simulink model "Continuous_Model"  (R2021b)
settings: Solver=VariableStepAuto  StartTime=0.0  StopTime=200.0  RelTol=1e-3
values from neighbouring files (symbols this model uses):
  mu0 = 0    [Continuous_Model_Parameters.m]
  n0 = 0    [Continuous_Model_Parameters.m]
  r0 = 0    [Continuous_Model_Parameters.m]
  s0 = 5    [Continuous_Model_Parameters.m]
  str0 = 0    [Continuous_Model_Parameters.m]
  T0 = 1    [Continuous_Model_Parameters.m]
  vx0 = 5    [Continuous_Model_Parameters.m]
  vy0 = 0    [Continuous_Model_Parameters.m]
libraries: dspsrcs4 x1
settings Model: Creator=21738394  LastModifiedBy=21738394

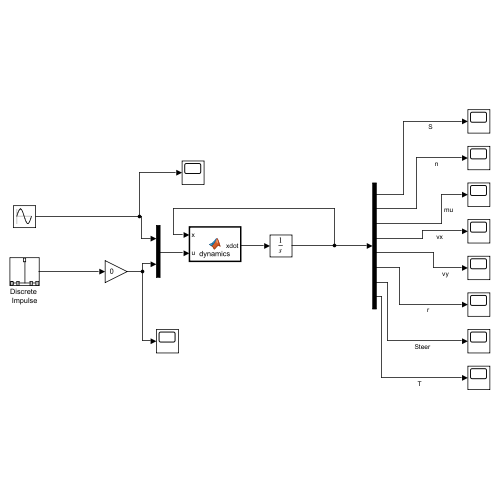
[thumbnail: Simulink's stored preview of the top-level diagram]
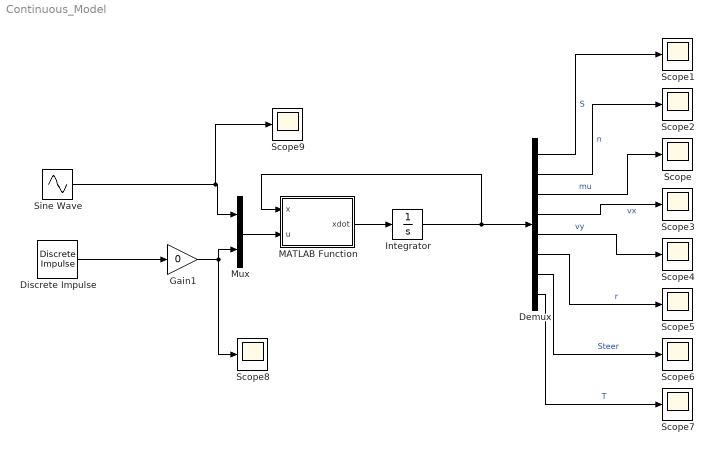
== system Continuous_Model ==
  Demux : Demux  Outputs=8
  Discrete Impulse : dspsrcs4/Discrete  Impulse  Delay=0  SampleTime=1  FrameSample=1  OutputFrames=off  dataType=double  isSigned=on  wordLen=16  udDataType=sfix(16)  fracBitsMode=Best precision  numFracBits=15  OutDataTypeStr=double  LastOutDataTypeStr=double
  Gain1 : Gain  Gain=0
  Integrator : Integrator  InitialCondition=[s0 n0 mu0 vx0 vy0 r0 str0 T0]
  MATLAB Function : MATLAB Function  TreatAsAtomicUnit=on
  Mux : Mux  Inputs=2
  Scope{,1..9} (10 alike) : Scope
  Sine Wave : Sin  Amplitude=(pi/(6*10))  Frequency=0.1  Phase=pi/2  SampleTime=0
  wires:
  Mux/1 -> MATLAB Function/2(u)
  MATLAB Function/1(xdot) -> Integrator/1
  Integrator/1 -> Demux/1, MATLAB Function/1(x)
  Demux/1 -> Scope1/1  "S"
  Demux/2 -> Scope2/1  "n"
  Demux/3 -> Scope/1  "mu"
  Demux/4 -> Scope3/1  "vx"
  Demux/5 -> Scope4/1  "vy"
  Demux/6 -> Scope5/1  "r"
  Demux/7 -> Scope6/1  "Steer"
  Demux/8 -> Scope7/1  "T"
  Gain1/1 -> Mux/2, Scope8/1
  Sine Wave/1 -> Scope9/1, Mux/1
  Discrete Impulse/1 -> Gain1/1

== matlab function Continuous_Model/MATLAB Function ==
  data: x input; u input; xdot output
 function xdot = dynamics(x,u)

s    = x(1);
n    = x(2);
mu   = x(3);
vx   = x(4);
vy   = x(5);
r    = x(6);
str  = x(7);
T    = x(8);


Delta_str   = u(1);
Delta_T     = u(2);

Ks = 0;

Bf = 10;
Br = 10;
Cf = 1.9;
Cr = 1.9;
Dr = 1;
Df = 1;
Cm = 5;
Cr0 = 0.0;
Cr2 = 0.2;
l_f = 0.15875;
l_r = 0.17145;
mass = 3.74;
Iz = 0.04712;
FN_r = (mass*9.81*l_r)/(l_r+l_f);
FN_f =(mass*9.81*l_f)/(l_r+l_f);
p_tv = 0;


Fx = (Cm*T) - Cr0 - (Cr2*(vx^2));
alpha_f = atan((vy + l_f*r)/vx) - str;
Fyf = FN_f*Df*sin(Cf*atan(Bf*alpha_f));
alpha_r = atan((vy - l_r*r)/vx) ;
Fyr = FN_r*Dr*sin(Cr*atan(Br*alpha_r));
Mtv = p_tv*(((tan(str)*vx)/(l_r + l_f)) - r);

sdot = ((vx*cos(mu)) - (vy*sin(mu)))/(1 - n*Ks);
ndot = (vx*sin(mu)) + (vy*cos(mu));
mudot = r - (Ks*sdot);
vxdot = (1/mass)*(Fx - Fyf*sin(str) + mass*vy*r);
vydot = (1/mass)*(Fyr + Fyr*cos(str) - mass*vx*r);
rdot = (1/Iz) * (Fyf*l_f*cos(str) - Fyr*l_r + Mtv)';

strdot = Delta_str;
Tdot = Delta_T;

xdot = [sdot ndot mudot vxdot vydot rdot strdot Tdot];
